simulink model "ModelSpeedSolver"  (R2019b)
settings: Solver=VariableStepAuto  StartTime=0.0  StopTime=1  RelTol=1e-3
values from neighbouring files (symbols this model uses):
  envFactor = struct    [inputSolver.m]
  X0 = 0/3.6    (= 0)    [inputSolver.m]
  Xfmax = 400/3.6    (= 111.111111111)    [inputSolver.m]
  Xfmin = 0/3.6    (= 0)    [inputSolver.m]
undefined symbols (not defined in the file or in its folder): modelPara, solverinput
settings Model: Creator=j9002  LastModifiedBy=j9002
settings DataIOCC: ReturnWorkspaceOutputs=off
settings DebuggingCC: ArithmeticOperatorsInVariantConditions=warning
settings SFSimCC: SimUseLocalCustomCode=off  CustomCodeUndefinedFunction=UseInterfaceOnly
settings RTWCC: RTWUseLocalCustomCode=off

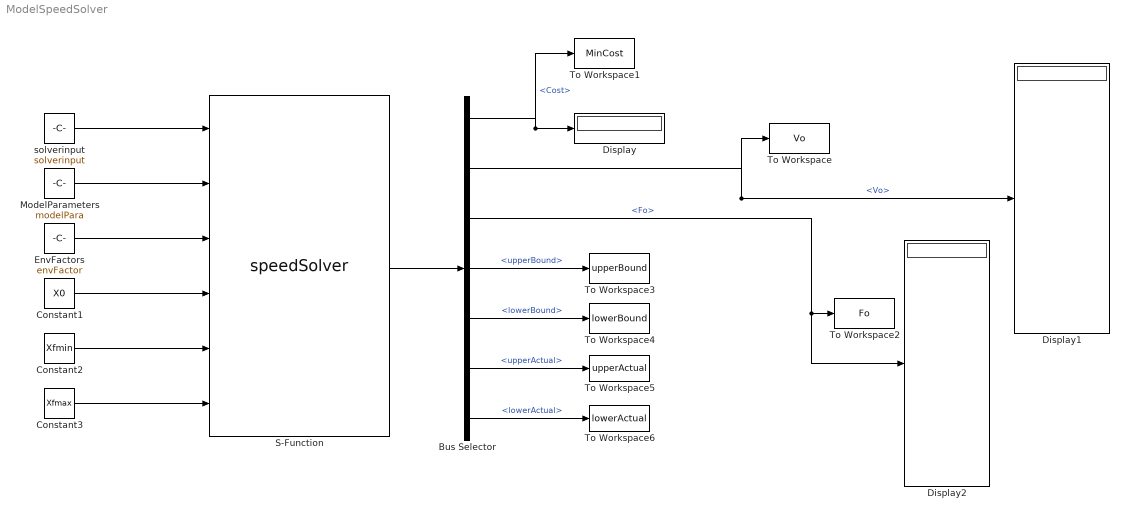
== system ModelSpeedSolver ==
  Bus Selector : BusSelector  OutputSignals=Cost,Vo,Fo,upperBound,lowerBound,upperActual,lowerActual
  Constant1 : Constant  Value=X0
  Constant2 : Constant  Value=Xfmin
  Constant3 : Constant  Value=Xfmax
  Display : Display
  Display1 : Display
  Display2 : Display
  EnvFactors : Constant  Value=envFactor  OutDataTypeStr=Bus: EnvFactor
  ModelParameters : Constant  Value=modelPara  OutDataTypeStr=Bus: SpeedDynParameter
  S-Function : S-Function  FunctionName=speedSolver  SFunctionDeploymentMode=off  EnableBusSupport=off
  To Workspace : ToWorkspace  VariableName=Vo  SampleTime=-1
  To Workspace1 : ToWorkspace  VariableName=MinCost  SampleTime=-1
  To Workspace2 : ToWorkspace  VariableName=Fo  SampleTime=-1
  To Workspace3 : ToWorkspace  VariableName=upperBound  SampleTime=-1
  To Workspace4 : ToWorkspace  VariableName=lowerBound  SampleTime=-1
  To Workspace5 : ToWorkspace  VariableName=upperActual  SampleTime=-1
  To Workspace6 : ToWorkspace  VariableName=lowerActual  SampleTime=-1
  solverinput : Constant  Value=solverinput  OutDataTypeStr=Bus: SolverInput
  wires:
  solverinput/1 -> S-Function/1
  ModelParameters/1 -> S-Function/2
  EnvFactors/1 -> S-Function/3
  Constant1/1 -> S-Function/4
  Constant2/1 -> S-Function/5
  Constant3/1 -> S-Function/6
  S-Function/1 -> Bus Selector/1
  Bus Selector/1 -> To Workspace1/1, Display/1  "<Cost>"
  Bus Selector/2 -> To Workspace/1, Display1/1  "<Vo>"
  Bus Selector/3 -> Display2/1, To Workspace2/1  "<Fo>"
  Bus Selector/4 -> To Workspace3/1  "<upperBound>"
  Bus Selector/5 -> To Workspace4/1  "<lowerBound>"
  Bus Selector/7 -> To Workspace6/1  "<lowerActual>"
  Bus Selector/6 -> To Workspace5/1  "<upperActual>"
